simulink model "test"  (R2016b)
settings: Solver=VariableStepAuto  StartTime=0.0  StopTime=50  RelTol=1e-3
undefined symbols (not defined in the file or in its folder): heading_error_conditioner
libraries: cstblocks x3, simulink_need_slupdate x1
settings Model: Creator=Zikinkeria  LastModifiedBy=Zikinkeria

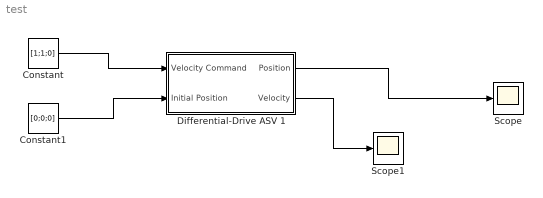
== system test ==
  Constant : Constant  Value=[1;1;0]
  Constant1 : Constant  Value=[0;0;0]
  Differential-Drive ASV 1 : Subsystem
  Scope : Scope
  Scope1 : Scope
  wires:
  Constant/1 -> Differential-Drive ASV 1/1(Velocity Command)
  Constant1/1 -> Differential-Drive ASV 1/2(Initial Position)
  Differential-Drive ASV 1/1(Position) -> Scope/1
  Differential-Drive ASV 1/2(Velocity) -> Scope1/1

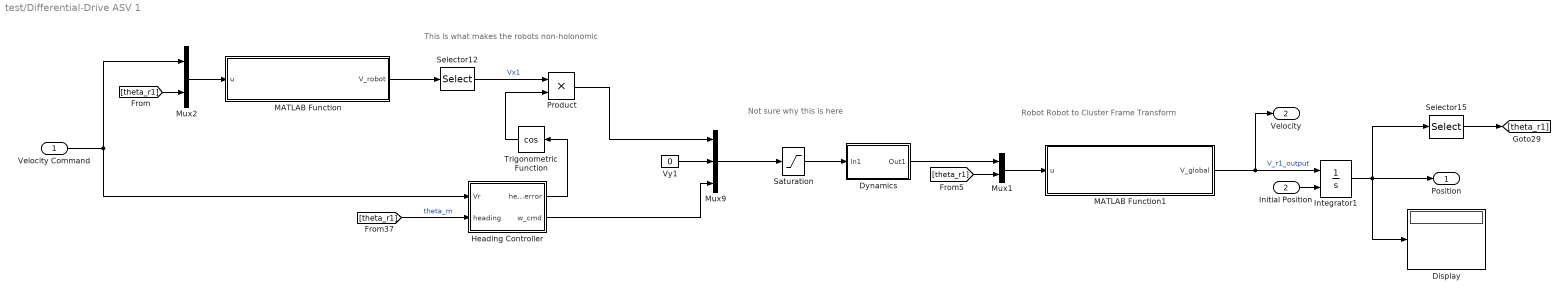
== system test/Differential-Drive ASV 1 ==
  note: Robot
      | Robot to Cluster
      | Frame Transform
  note: Not sure
      | why this is here
  note: This is what makes the robots non-holonomic
  Velocity Command : Inport
  Initial Position : Inport  Port=2
  Display : Display
  Dynamics : Subsystem
  Heading Controller : Subsystem
  Integrator1 : Integrator  InitialConditionSource=external
  MATLAB Function : MATLAB Function  TreatAsAtomicUnit=on
  MATLAB Function1 : MATLAB Function  TreatAsAtomicUnit=on
  Mux1 : Mux  Inputs=2
  Mux2 : Mux  Inputs=2
  Mux9 : Mux  Inputs=3
  Product : Product  RndMeth=Zero
  Saturation : Saturate  UpperLimit=10  LowerLimit=-10
  Selector12 : Selector  InputPortWidth=3  IndexOptions=Index vector (dialog)  Indices=[1]  OutputSizes=1
  Selector15 : Selector  InputPortWidth=3  IndexOptions=Index vector (dialog)  Indices=[3]  OutputSizes=1
  Trigonometric Function : Trigonometry  Operator=cos
  Vy1 : Constant  Value=0
  Position : Outport
  Velocity : Outport  Port=2
  wires:
  Trigonometric Function/1 -> Product/2
  Mux9/1 -> Saturation/1
  Saturation/1 -> Dynamics/1(In1)
  Selector15/1 -> [theta_r1]
  [theta_r1] -> Mux1/2
  Vy1/1 -> Mux9/2
  Selector12/1 -> Product/1  "Vx1"
  [theta_r1] -> Mux2/2
  MATLAB Function/1(V_robot) -> Selector12/1
  Dynamics/1(Out1) -> Mux1/1
  MATLAB Function1/1(V_global) -> Integrator1/1, Velocity/1  "V_r1_output"
  Integrator1/1 -> Selector15/1, Position/1, Display/1
  Initial Position/1 -> Integrator1/2
  Product/1 -> Mux9/1
  Mux2/1 -> MATLAB Function/1(u)
  Mux1/1 -> MATLAB Function1/1(u)
  Velocity Command/1 -> Mux2/1, Heading Controller/1(Vr)
  [theta_r1] -> Heading Controller/2(heading)  "theta_m"
  Heading Controller/1(heading error) -> Trigonometric Function/1
  Heading Controller/2(w_cmd) -> Mux9/3

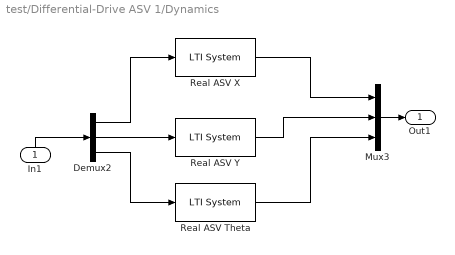
== system test/Differential-Drive ASV 1/Dynamics ==
  In1 : Inport
  Demux2 : Demux  Outputs=3
  Mux3 : Mux  Inputs=3
  Real ASV Theta : cstblocks/LTI System  sys=tf(1,[1.2 1])  IC=[]
  Real ASV X : cstblocks/LTI System  sys=tf(1,[1.5 1])  IC=[]
  Real ASV Y : cstblocks/LTI System  sys=tf(1,[4 1])  IC=[]
  Out1 : Outport
  wires:
  Mux3/1 -> Out1/1
  In1/1 -> Demux2/1
  Demux2/1 -> Real ASV X/1
  Demux2/2 -> Real ASV Y/1
  Demux2/3 -> Real ASV Theta/1
  Real ASV X/1 -> Mux3/1
  Real ASV Y/1 -> Mux3/2
  Real ASV Theta/1 -> Mux3/3

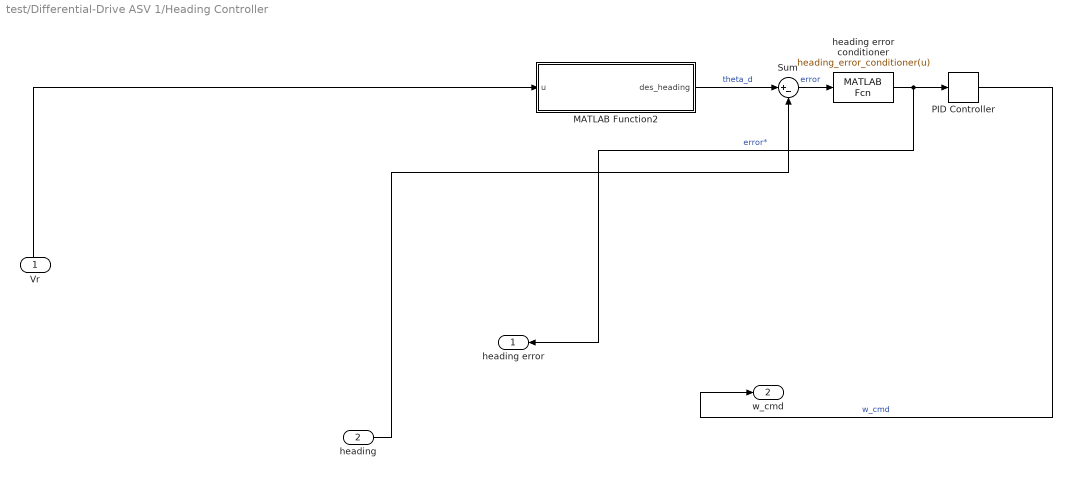
== system test/Differential-Drive ASV 1/Heading Controller ==
  Vr : Inport
  heading : Inport  Port=2
  MATLAB Function2 : MATLAB Function  TreatAsAtomicUnit=on
  PID Controller : simulink_need_slupdate/PID Controller  P=1  I=0  D=0
  Sum : Sum  Inputs=|+-
  heading error conditioner : MATLABFcn  MATLABFcn=heading_error_conditioner(u)
  heading error : Outport
  w_cmd : Outport  Port=2
  wires:
  MATLAB Function2/1(des_heading) -> Sum/1  "theta_d"
  heading/1 -> Sum/2
  PID Controller/1 -> w_cmd/1  "w_cmd"
  heading error conditioner/1 -> heading error/1, PID Controller/1  "error*"
  Sum/1 -> heading error conditioner/1  "error"
  Vr/1 -> MATLAB Function2/1(u)

== matlab function test/Differential-Drive ASV 1/Heading Controller/MATLAB Function2 ==
  data: u input; des_heading output
function des_heading = get_heading_angle_from_vel(u)
%This function computes the heading angle for a differential drive based on the cluster velocities of robots
%threshold is the min vel that outputs a desired heading, otherwise is zero.
%arguments:     u = [Vx Vy threshold]
%output:     output = [theta_des]
%Initialize variables
Vx = u(1);
Vy = u(2);
% positive heading is in clockwise direction measured from global y
des_heading=atan2(Vy,Vx);  %desires heading based on commanded velocity vector, in global frame.
end

== matlab function test/Differential-Drive ASV 1/MATLAB Function ==
  data: u input; V_robot output
function V_robot = Global_to_Robot_Transformation(u)
%This function calculates the local robot velocities
%based on the global robot velocities

%Initialize Variables
V_global = [u(1);u(2);u(3)];
theta = u(4);

T = [cos(theta) sin(theta) 0;...
    -sin(theta) cos(theta) 0;...
    0               0       1]; % postive Z is up so theta is counter clockwise
%    0               0           -1]; % -1 means clockwise around z is positive 
V_robot = T*V_global;

== matlab function test/Differential-Drive ASV 1/MATLAB Function1 ==
  data: u input; V_global output
function V_global = Robot_to_Global_Transformation(u)
%This function calculates the local robot velocities
%based on the global robot velocities

%Initialize Variables
V_robot = [u(1);u(2);u(3)];
theta = u(4);

T = [cos(theta) -sin(theta) 0;...
    sin(theta) cos(theta) 0;...
    0               0           1]';
V_global = T*V_robot;
